simulink model "prob1"  (R2015a)
settings: Solver=ode4  StartTime=0.0  StopTime=10.0  RelTol=1e-3
settings Model: Creator=Aranya Dan  LastModifiedBy=Aranya Dan

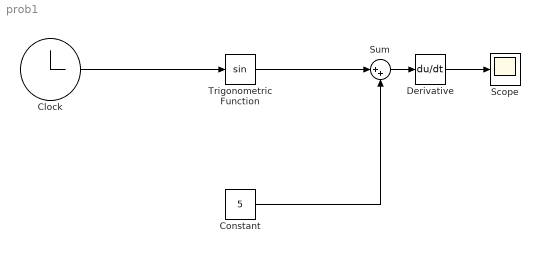
== system prob1 ==
  Clock : Clock
  Constant : Constant  Value=5
  Derivative : Derivative
  Scope : Scope
  Sum : Sum  Inputs=|++
  Trigonometric Function : Trigonometry
  wires:
  Clock/1 -> Trigonometric Function/1
  Trigonometric Function/1 -> Sum/1
  Constant/1 -> Sum/2
  Sum/1 -> Derivative/1
  Derivative/1 -> Scope/1
